simulink model "PIDClosedLoop"  (R2024b)
settings: Solver=VariableStepAuto  StartTime=0.0  StopTime=10.0  RelTol=1e-3
settings Model: Creator=arunk  LastModifiedBy=arunk

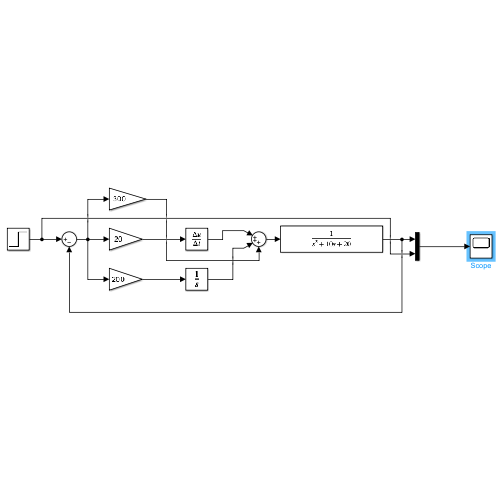
[thumbnail: Simulink's stored preview of the top-level diagram]
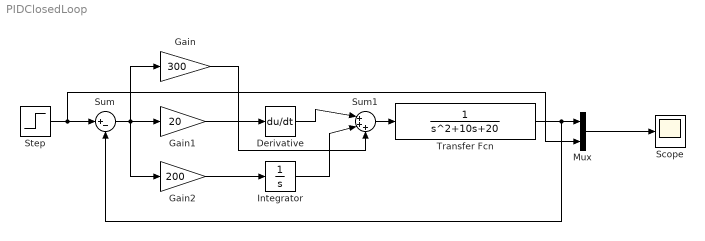
== system PIDClosedLoop ==
  Derivative : Derivative
  Gain : Gain  Gain=300
  Gain1 : Gain  Gain=20
  Gain2 : Gain  Gain=200
  Integrator : Integrator
  Mux : Mux  Inputs=2
  Scope : Scope
  Step : Step  SampleTime=0
  Sum : Sum  Inputs=|+-
  Sum1 : Sum  Inputs=|+++
  Transfer Fcn : TransferFcn  Denominator=[1 10 20]
  wires:
  Sum/1 -> Gain2/1, Gain/1, Gain1/1
  Gain2/1 -> Integrator/1
  Gain1/1 -> Derivative/1
  Derivative/1 -> Sum1/1
  Integrator/1 -> Sum1/2
  Gain/1 -> Sum1/3
  Sum1/1 -> Transfer Fcn/1
  Step/1 -> Mux/2, Sum/1
  Mux/1 -> Scope/1
  Transfer Fcn/1 -> Sum/2, Mux/1
